simulink model "HLC_test_2018"  (R2020a)
settings: Solver=VariableStepAuto  StartTime=0.0  StopTime=10.0  RelTol=1e-3
values from neighbouring files (symbols this model uses):
  Ignition = timeseries    [TT1_in.m]
undefined symbols (not defined in the file or in its folder): Ambiant_Angle, DN, Light, Lock, Road_T, Speed_InKMPH, V_Detected, Weather
libraries: simulink x59
settings Model: Creator=VIJAY BANDEPPA MURGE  LastModifiedBy=VIJAY BANDEPPA MURGE
settings DebuggingCC: ArithmeticOperatorsInVariantConditions=warning
settings SFSimCC: CustomCodeUndefinedFunction=UseInterfaceOnly

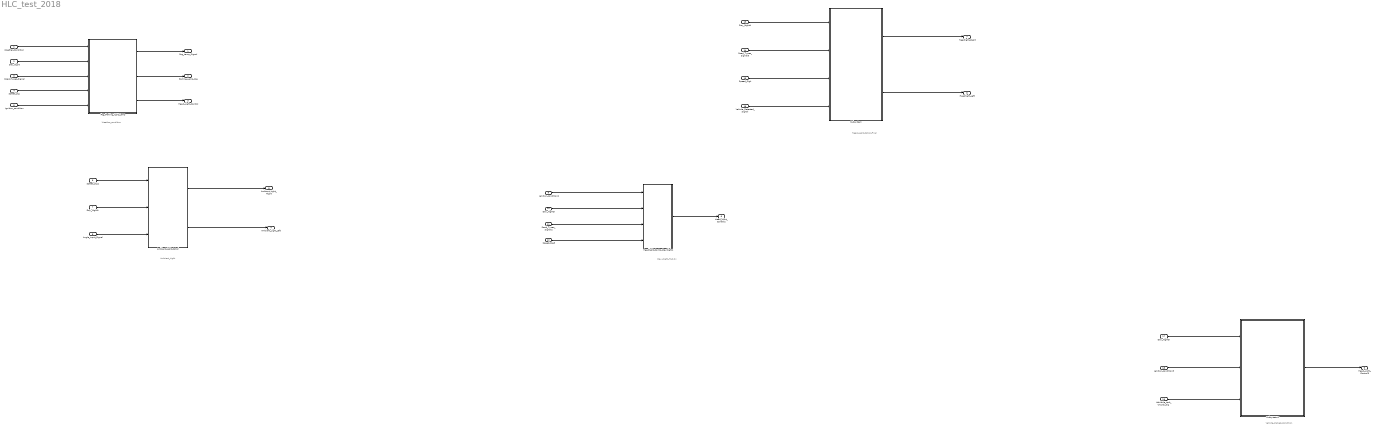
== system HLC_test_2018 ==
  note: Ambient_Light
  note: Day_Night_HLC.slx
  note: Head_Light_Cotrol_Final
  note: Vehicle_Parked_Condition
  note: Weather_condition
  Weather_Condition : Inport
  Day_Night : Inport  Port=2
  Road_Types_Signal : Inport  Port=3
  Speed_Sig : Inport  Port=4
  Ignition_condition : Inport  Port=5
  Speed_Sig1 : Inport  Port=6
  Day_Night1 : Inport  Port=7
  Angle_Input_Signal : Inport  Port=8
  Ignition_condition2 : Inport  Port=9
  Day_Night3 : Inport  Port=10
  Road_Types_Signal2 : Inport  Port=11
  Speed_Sig3 : Inport  Port=12
  Day_Night4 : Inport  Port=13
  Road_Types_Signal3 : Inport  Port=14
  Speed_Sig4 : Inport  Port=15
  Vehicle_Detected_Signal : Inport  Port=16
  Day_Night5 : Inport  Port=17
  Ignition_condition3 : Inport  Port=18
  Vehichle_Lock_UnLock_Sig : Inport  Port=19
  Ambient_Light_Cotrol : Subsystem  Description=This System is use for cotrol abbiant Light Of cars and other havey loded vehicles
  Fog_Parking_light_Lamp : Subsystem  Description=Cotrol of Fog lamp_Parking Light and hedlight in differant modes
  Headlight_Contro_DayNight1 : Subsystem  Description=testing_dayNight_Control of the cars
  Subsystem : Subsystem
  Subsystem2 : Subsystem
  Fog_Lamp_Signal : Outport
  Parking_Lamp_Sig : Outport  Port=2
  Head_Light_Control : Outport  Port=3
  Ambiant_Light_Left : Outport  Port=4
  Ambiant_Light_Right : Outport  Port=5
  Head_Light_Control2 : Outport  Port=6
  Headlight_Right : Outport  Port=7
  Headlight_Left : Outport  Port=8
  Head_Light_Control3 : Outport  Port=9
  wires:
  Fog_Parking_light_Lamp/3(Head_Light_Control) -> Head_Light_Control/1
  Ignition_condition/1 -> Fog_Parking_light_Lamp/5(Ignition_condition)  "Ignition_condition"
  Fog_Parking_light_Lamp/2(Parking_Lamp_Sig) -> Parking_Lamp_Sig/1
  Weather_Condition/1 -> Fog_Parking_light_Lamp/1(Weather_Condition)  "Weather_Condition"
  Fog_Parking_light_Lamp/1(Fog_Lamp_Signal) -> Fog_Lamp_Signal/1
  Speed_Sig/1 -> Fog_Parking_light_Lamp/4(Speed_Sig)  "Speed_Sig"
  Day_Night/1 -> Fog_Parking_light_Lamp/2(Day_Night)  "Day_Night"
  Road_Types_Signal/1 -> Fog_Parking_light_Lamp/3(Road_Types_Signal)  "Road_Types_Signal"
  Day_Night1/1 -> Ambient_Light_Cotrol/2(Day_Night)  "Day_Night"
  Ambient_Light_Cotrol/1(Ambiant_Light_Right) -> Ambiant_Light_Right/1
  Angle_Input_Signal/1 -> Ambient_Light_Cotrol/3(Angle_Input_Signal)  "Angle_Input_Signal"
  Speed_Sig1/1 -> Ambient_Light_Cotrol/1(Speed_Sig)  "Speed_Sig"
  Ambient_Light_Cotrol/2(Ambiant_Light_Left) -> Ambiant_Light_Left/1
  Ignition_condition2/1 -> Headlight_Contro_DayNight1/1(Ignition_condition)  "Ignition_condition"
  Day_Night3/1 -> Headlight_Contro_DayNight1/2(Day_Night)  "Day_Night"
  Speed_Sig3/1 -> Headlight_Contro_DayNight1/4(Speed_Sig)  "Speed_Sig"
  Headlight_Contro_DayNight1/1(Head_Light_Control) -> Head_Light_Control2/1
  Road_Types_Signal2/1 -> Headlight_Contro_DayNight1/3(Road_Types_Signal)  "Road_Types_Signal"
  Speed_Sig4/1 -> Subsystem/3(Speed_Sig)  "Speed_Sig"
  Road_Types_Signal3/1 -> Subsystem/2(Road_Types_Signal)  "Road_Types_Signal"
  Vehicle_Detected_Signal/1 -> Subsystem/4(Vehicle_Detected_Signal)  "Vehicle_Detected_Signal"
  Subsystem/1(Headlight_Right) -> Headlight_Right/1
  Subsystem/2(Headlight_Left) -> Headlight_Left/1
  Day_Night4/1 -> Subsystem/1(Day_Night)  "Day_Night"
  Subsystem2/1(Head_Light_Control) -> Head_Light_Control3/1
  Vehichle_Lock_UnLock_Sig/1 -> Subsystem2/3(Vehichle_Lock_UnLock_Sig)  "Vehichle_Lock_UnLock_Sig"
  Ignition_condition3/1 -> Subsystem2/2(Ignition_condition)  "Ignition_condition"
  Day_Night5/1 -> Subsystem2/1(Day_Night)  "Day_Night"

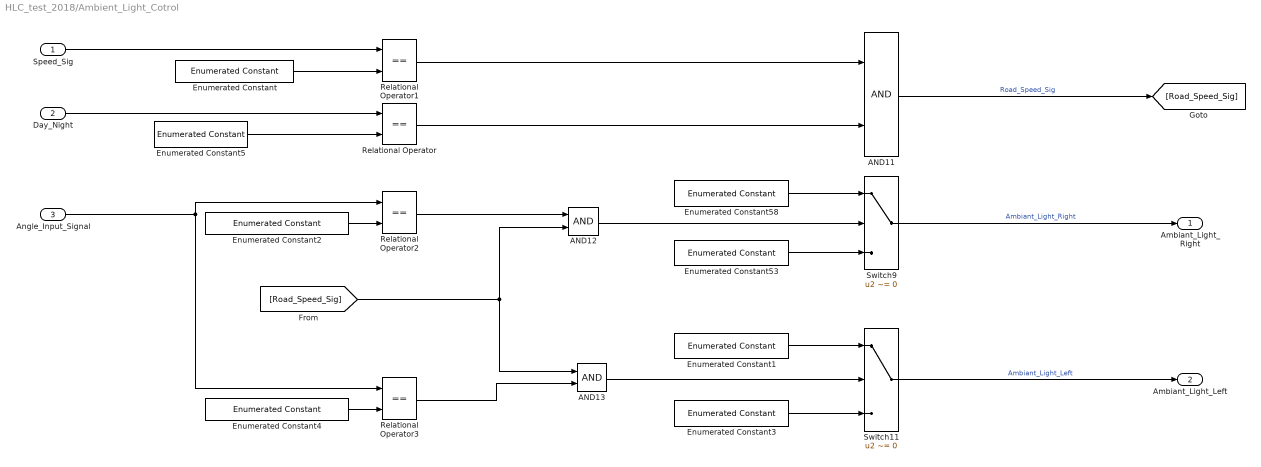
== system HLC_test_2018/Ambient_Light_Cotrol ==
  Speed_Sig : Inport
  Day_Night : Inport  Port=2
  Angle_Input_Signal : Inport  Port=3
  AND11 : Logic  AllPortsSameDT=off
  AND12 : Logic  AllPortsSameDT=off
  AND13 : Logic  AllPortsSameDT=off
  Enumerated Constant : simulink/Sources/Enumerated Constant  OutDataTypeStr=Enum: Speed_InKMPH  Value=Speed_InKMPH.Speed_Value  SampleTime=inf
  Enumerated Constant1 : simulink/Sources/Enumerated Constant  OutDataTypeStr=Enum: Light  Value=Light.L_Ambient_Light_On  SampleTime=inf
  Enumerated Constant2 : simulink/Sources/Enumerated Constant  OutDataTypeStr=Enum: Ambiant_Angle  Value=Ambiant_Angle.Ambiant_RHS_Angle  SampleTime=inf
  Enumerated Constant3 : simulink/Sources/Enumerated Constant  OutDataTypeStr=Enum: Light  Value=Light.L_Ambient_Light_off  SampleTime=inf
  Enumerated Constant4 : simulink/Sources/Enumerated Constant  OutDataTypeStr=Enum: Ambiant_Angle  Value=Ambiant_Angle.Ambiant_LHS_Angle  SampleTime=inf
  Enumerated Constant5 : simulink/Sources/Enumerated Constant  OutDataTypeStr=Enum: DN  Value=DN.Darkness  SampleTime=inf
  Enumerated Constant53 : simulink/Sources/Enumerated Constant  OutDataTypeStr=Enum: Light  Value=Light.R_Ambient_Light_off  SampleTime=inf
  Enumerated Constant58 : simulink/Sources/Enumerated Constant  OutDataTypeStr=Enum: Light  Value=Light.R_Ambient_Light_On  SampleTime=inf
  Relational Operator : RelationalOperator  Operator===  OutDataTypeStr=boolean  RndMeth=Simplest
  Relational Operator1 : RelationalOperator  Operator===  OutDataTypeStr=boolean  RndMeth=Simplest
  Relational Operator2 : RelationalOperator  Operator===  OutDataTypeStr=boolean  RndMeth=Simplest
  Relational Operator3 : RelationalOperator  Operator===  RndMeth=Simplest
  Switch11 : Switch  Criteria=u2 ~= 0  OutDataTypeStr=Inherit: Inherit via back propagation
  Switch9 : Switch  Criteria=u2 ~= 0  OutDataTypeStr=Inherit: Inherit via back propagation
  Ambiant_Light_Right : Outport
  Ambiant_Light_Left : Outport  Port=2
  wires:
  Enumerated Constant5/1 -> Relational Operator/2
  [Road_Speed_Sig] -> AND12/2, AND13/1
  Angle_Input_Signal/1 -> Relational Operator2/1, Relational Operator3/1
  Relational Operator3/1 -> AND13/2
  AND11/1 -> [Road_Speed_Sig]  "Road_Speed_Sig"
  AND12/1 -> Switch9/2
  Enumerated Constant1/1 -> Switch11/1
  AND13/1 -> Switch11/2
  Enumerated Constant58/1 -> Switch9/1
  Relational Operator2/1 -> AND12/1
  Relational Operator/1 -> AND11/2
  Enumerated Constant53/1 -> Switch9/3
  Enumerated Constant3/1 -> Switch11/3
  Day_Night/1 -> Relational Operator/1
  Switch9/1 -> Ambiant_Light_Right/1  "Ambiant_Light_Right"
  Switch11/1 -> Ambiant_Light_Left/1  "Ambiant_Light_Left"
  Speed_Sig/1 -> Relational Operator1/1
  Enumerated Constant/1 -> Relational Operator1/2
  Relational Operator1/1 -> AND11/1
  Enumerated Constant2/1 -> Relational Operator2/2
  Enumerated Constant4/1 -> Relational Operator3/2

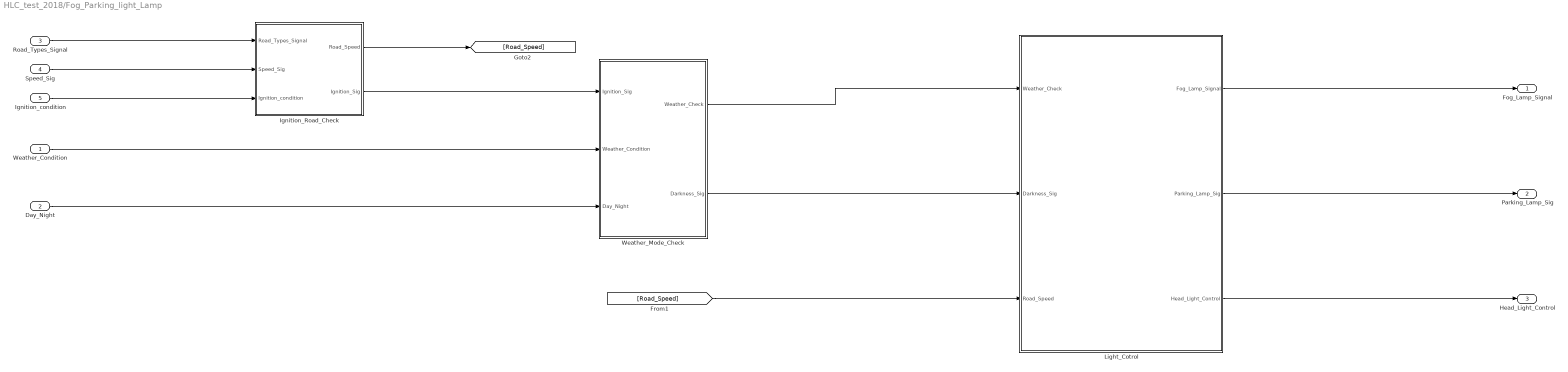
== system HLC_test_2018/Fog_Parking_light_Lamp ==
  Weather_Condition : Inport
  Day_Night : Inport  Port=2
  Road_Types_Signal : Inport  Port=3
  Speed_Sig : Inport  Port=4
  Ignition_condition : Inport  Port=5
  Ignition_Road_Check : Subsystem  Description=ignition and Road_Check
  Light_Cotrol : Subsystem  Description=it control the fog parking and head light
  Weather_Mode_Check : Subsystem  Description=it check weather and raod conditions
  Fog_Lamp_Signal : Outport
  Parking_Lamp_Sig : Outport  Port=2
  Head_Light_Control : Outport  Port=3
  wires:
  Weather_Condition/1 -> Weather_Mode_Check/2(Weather_Condition)
  Ignition_Road_Check/2(Ignition_Sig) -> Weather_Mode_Check/1(Ignition_Sig)
  Day_Night/1 -> Weather_Mode_Check/3(Day_Night)
  Road_Types_Signal/1 -> Ignition_Road_Check/1(Road_Types_Signal)
  Speed_Sig/1 -> Ignition_Road_Check/2(Speed_Sig)
  Ignition_condition/1 -> Ignition_Road_Check/3(Ignition_condition)
  Ignition_Road_Check/1(Road_Speed) -> [Road_Speed]
  Weather_Mode_Check/1(Weather_Check) -> Light_Cotrol/1(Weather_Check)
  Weather_Mode_Check/2(Darkness_Sig) -> Light_Cotrol/2(Darkness_Sig)
  Light_Cotrol/1(Fog_Lamp_Signal) -> Fog_Lamp_Signal/1
  Light_Cotrol/2(Parking_Lamp_Sig) -> Parking_Lamp_Sig/1
  Light_Cotrol/3(Head_Light_Control) -> Head_Light_Control/1
  [Road_Speed] -> Light_Cotrol/3(Road_Speed)

== system HLC_test_2018/Headlight_Contro_DayNight1 ==
  Ignition_condition : Inport
  Day_Night : Inport  Port=2
  Road_Types_Signal : Inport  Port=3
  Speed_Sig : Inport  Port=4
  Day_Ignition_Check : Subsystem  Description=check road and ignition condition
  Road_Syateam : Subsystem  Description=Road check condition
  Head_Light_Control : Outport
  wires:
  Road_Types_Signal/1 -> Road_Syateam/1(Road_Types_Signal)
  Speed_Sig/1 -> Road_Syateam/2(Speed_Sig)
  Ignition_condition/1 -> Day_Ignition_Check/1(Ignition_condition)
  Day_Night/1 -> Day_Ignition_Check/2(Day_Night)
  Day_Ignition_Check/1(Head_Light_Control) -> Head_Light_Control/1
  Road_Syateam/1(Road_Speed_Signal_Check) -> Day_Ignition_Check/3(Road_Speed_Signal_Check)

== system HLC_test_2018/Subsystem ==
  Day_Night : Inport
  Road_Types_Signal : Inport  Port=2
  Speed_Sig : Inport  Port=3
  Vehicle_Detected_Signal : Inport  Port=4
  Head_Light_Cotrol : Subsystem
  RHS_LHS_Vehicle_Detct : Subsystem
  Road_Vehicle_Dect : Subsystem
  Headlight_Right : Outport
  Headlight_Left : Outport  Port=2
  wires:
  Road_Types_Signal/1 -> Road_Vehicle_Dect/1(Road_Types_Signal)
  Speed_Sig/1 -> Road_Vehicle_Dect/2(Speed_Sig)
  Vehicle_Detected_Signal/1 -> RHS_LHS_Vehicle_Detct/1(Vehicle_Detected_Signal), Road_Vehicle_Dect/3(Vehicle_Detected_Signal)
  [Day_Night] -> RHS_LHS_Vehicle_Detct/2(Day_Night)
  Day_Night/1 -> [Day_Night], Head_Light_Cotrol/1(Day_Night)
  Road_Vehicle_Dect/1(Road_Vehical_Signal) -> Head_Light_Cotrol/2(Road_Vehical_Signal)
  RHS_LHS_Vehicle_Detct/1(Right_Vehicle_Detected) -> Head_Light_Cotrol/3(Right_Vehicle_Detected)
  RHS_LHS_Vehicle_Detct/2(Left_Vehicle_Detected) -> Head_Light_Cotrol/4(Left_Vehicle_Detected)
  Head_Light_Cotrol/1(Headlight_Right) -> Headlight_Right/1
  Head_Light_Cotrol/2(Headlight_Left) -> Headlight_Left/1

== system HLC_test_2018/Subsystem2 ==
  Day_Night : Inport
  Ignition_condition : Inport  Port=2
  Vehichle_Lock_UnLock_Sig : Inport  Port=3
  Subsystem : Subsystem
  Subsystem1 : Subsystem
  Head_Light_Control : Outport
  wires:
  Subsystem/5(Lock_Sig) -> Subsystem1/5(Lock_Sig)
  Subsystem/4(Ignition_sig) -> Subsystem1/4(Ignition_sig)
  Subsystem/1(Day_Night_Sig) -> Subsystem1/1(Day_Night_Sig)
  Subsystem/2(Day_Ign_Lock_Sig) -> Subsystem1/2(Day_Ign_Lock_Sig)
  Subsystem/3(Darkness_Sig) -> Subsystem1/3(Darkness_Sig)
  Day_Night/1 -> Subsystem/1(Day_Night)
  Subsystem1/1(Head_Light_Control) -> Head_Light_Control/1
  Ignition_condition/1 -> Subsystem/2(Ignition_condition)
  Vehichle_Lock_UnLock_Sig/1 -> Subsystem/3(Vehichle_Lock_UnLock_Sig)

== system HLC_test_2018/Fog_Parking_light_Lamp/Ignition_Road_Check ==
  Road_Types_Signal : Inport
  Speed_Sig : Inport  Port=2
  Ignition_condition : Inport  Port=3
  AND9 : Logic  Inputs=3  AllPortsSameDT=off  OutDataTypeStr=boolean
  Compare To Constant : simulink/Logic and Bit Operations/Compare To Constant  relop=<=  const=3.0  OutDataTypeStr=boolean
  Enumerated Constant54 : simulink/Sources/Enumerated Constant  OutDataTypeStr=Enum: Ignition  Value=Ignition.Ignition_On  SampleTime=inf
  Enumerated Constant6 : simulink/Sources/Enumerated Constant  OutDataTypeStr=Enum: Road_T  Value=Road_T.Inside_City_Road  SampleTime=inf
  Relational Operator1 : RelationalOperator  Operator=~=  OutDataTypeStr=boolean  RndMeth=Simplest
  Relational Operator18 : RelationalOperator  Operator===  OutDataTypeStr=boolean  RndMeth=Simplest
  Road_Speed : Outport
  Ignition_Sig : Outport  Port=2
  wires:
  Enumerated Constant6/1 -> Relational Operator1/2
  Relational Operator18/1 -> Ignition_Sig/1, AND9/3  "Ignition_Sig"
  Relational Operator1/1 -> AND9/1
  Enumerated Constant54/1 -> Relational Operator18/2
  Compare To Constant/1 -> AND9/2
  AND9/1 -> Road_Speed/1  "Road_Speed"
  Speed_Sig/1 -> Compare To Constant/1
  Road_Types_Signal/1 -> Relational Operator1/1
  Ignition_condition/1 -> Relational Operator18/1

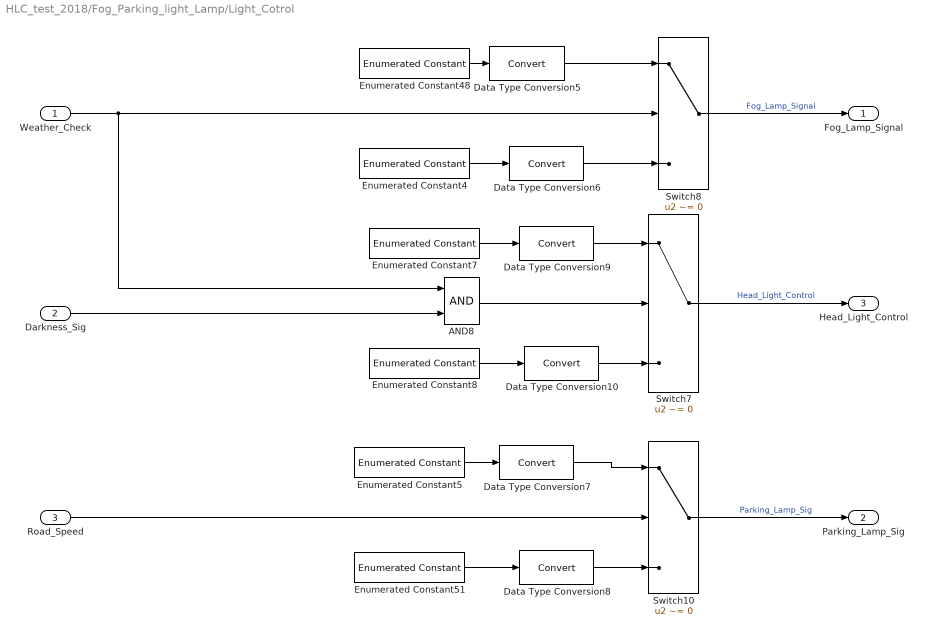
== system HLC_test_2018/Fog_Parking_light_Lamp/Light_Cotrol ==
  Weather_Check : Inport
  Darkness_Sig : Inport  Port=2
  Road_Speed : Inport  Port=3
  AND8 : Logic  AllPortsSameDT=off  OutDataTypeStr=boolean
  Data Type Conversion{5..10} (6 alike) : DataTypeConversion
  Enumerated Constant4 : simulink/Sources/Enumerated Constant  OutDataTypeStr=Enum: Light  Value=Light.Fog_Lamp_off  SampleTime=inf
  Enumerated Constant48 : simulink/Sources/Enumerated Constant  OutDataTypeStr=Enum: Light  Value=Light.Fog_Lamp_ON  SampleTime=inf
  Enumerated Constant5 : simulink/Sources/Enumerated Constant  OutDataTypeStr=Enum: Light  Value=Light.Parking_Light_On  SampleTime=inf
  Enumerated Constant51 : simulink/Sources/Enumerated Constant  OutDataTypeStr=Enum: Light  Value=Light.Parking_Light_Off  SampleTime=inf
  Enumerated Constant7 : simulink/Sources/Enumerated Constant  OutDataTypeStr=Enum: Light  Value=Light.Low_Beam  SampleTime=inf
  Enumerated Constant8 : simulink/Sources/Enumerated Constant  OutDataTypeStr=Enum: Light  Value=Light.Headlight_Off  SampleTime=inf
  Switch10 : Switch  Criteria=u2 ~= 0  OutDataTypeStr=Inherit: Inherit via back propagation
  Switch7 : Switch  Criteria=u2 ~= 0  OutDataTypeStr=Inherit: Inherit via back propagation
  Switch8 : Switch  Criteria=u2 ~= 0  OutDataTypeStr=Inherit: Inherit via back propagation
  Fog_Lamp_Signal : Outport
  Parking_Lamp_Sig : Outport  Port=2
  Head_Light_Control : Outport  Port=3
  wires:
  Enumerated Constant48/1 -> Data Type Conversion5/1
  Enumerated Constant51/1 -> Data Type Conversion8/1
  Data Type Conversion10/1 -> Switch7/3
  Data Type Conversion7/1 -> Switch10/1
  AND8/1 -> Switch7/2
  Data Type Conversion9/1 -> Switch7/1
  Enumerated Constant4/1 -> Data Type Conversion6/1
  Data Type Conversion5/1 -> Switch8/1
  Enumerated Constant8/1 -> Data Type Conversion10/1
  Enumerated Constant7/1 -> Data Type Conversion9/1
  Data Type Conversion8/1 -> Switch10/3
  Enumerated Constant5/1 -> Data Type Conversion7/1
  Data Type Conversion6/1 -> Switch8/3
  Weather_Check/1 -> AND8/1, Switch8/2
  Road_Speed/1 -> Switch10/2
  Switch10/1 -> Parking_Lamp_Sig/1  "Parking_Lamp_Sig"
  Switch8/1 -> Fog_Lamp_Signal/1  "Fog_Lamp_Signal"
  Darkness_Sig/1 -> AND8/2
  Switch7/1 -> Head_Light_Control/1  "Head_Light_Control"

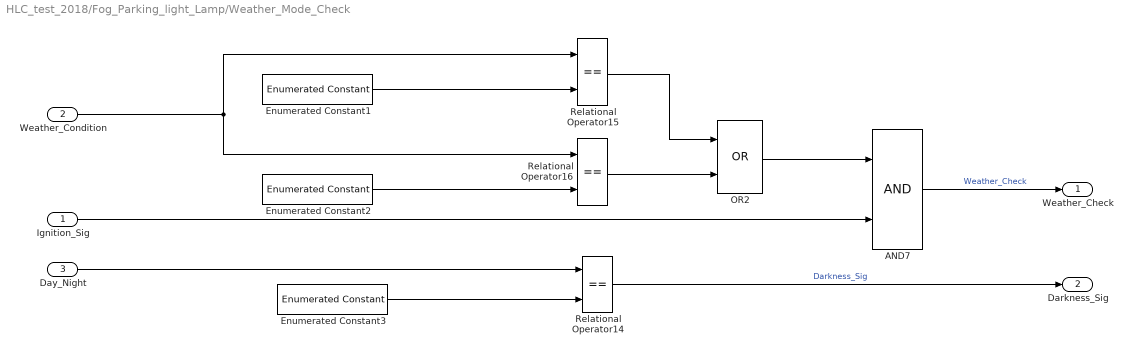
== system HLC_test_2018/Fog_Parking_light_Lamp/Weather_Mode_Check ==
  Ignition_Sig : Inport
  Weather_Condition : Inport  Port=2
  Day_Night : Inport  Port=3
  AND7 : Logic  AllPortsSameDT=off  OutDataTypeStr=boolean
  Enumerated Constant1 : simulink/Sources/Enumerated Constant  OutDataTypeStr=Enum: Weather  Value=Weather.Fog_Detected  SampleTime=inf
  Enumerated Constant2 : simulink/Sources/Enumerated Constant  OutDataTypeStr=Enum: Weather  Value=Weather.Rain_Detected  SampleTime=inf
  Enumerated Constant3 : simulink/Sources/Enumerated Constant  OutDataTypeStr=Enum: DN  Value=DN.Darkness  SampleTime=inf
  OR2 : Logic  Operator=OR  AllPortsSameDT=off  OutDataTypeStr=boolean
  Relational Operator14 : RelationalOperator  Operator===  OutDataTypeStr=boolean  RndMeth=Simplest
  Relational Operator15 : RelationalOperator  Operator===  OutDataTypeStr=boolean  RndMeth=Simplest
  Relational Operator16 : RelationalOperator  Operator===  OutDataTypeStr=boolean  RndMeth=Simplest
  Weather_Check : Outport
  Darkness_Sig : Outport  Port=2
  wires:
  Ignition_Sig/1 -> AND7/2
  Enumerated Constant2/1 -> Relational Operator16/2
  Weather_Condition/1 -> Relational Operator15/1, Relational Operator16/1
  Enumerated Constant3/1 -> Relational Operator14/2
  Enumerated Constant1/1 -> Relational Operator15/2
  Relational Operator15/1 -> OR2/1
  OR2/1 -> AND7/1
  Relational Operator16/1 -> OR2/2
  AND7/1 -> Weather_Check/1  "Weather_Check"
  Day_Night/1 -> Relational Operator14/1
  Relational Operator14/1 -> Darkness_Sig/1  "Darkness_Sig"

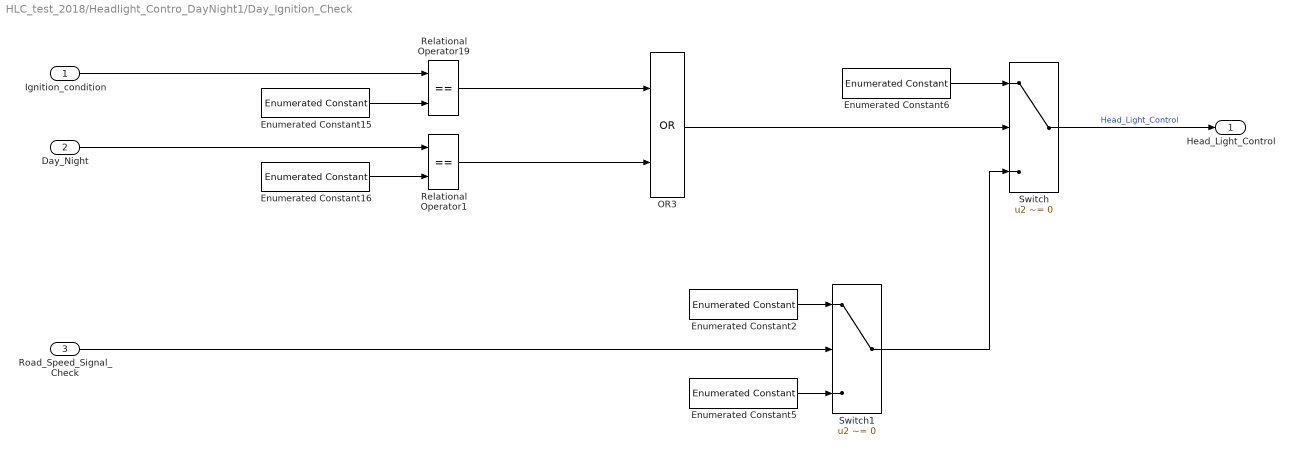
== system HLC_test_2018/Headlight_Contro_DayNight1/Day_Ignition_Check ==
  Ignition_condition : Inport
  Day_Night : Inport  Port=2
  Road_Speed_Signal_Check : Inport  Port=3
  Enumerated Constant15 : simulink/Sources/Enumerated Constant  OutDataTypeStr=Enum: Ignition  Value=Ignition.Ignition_Off  SampleTime=inf
  Enumerated Constant16 : simulink/Sources/Enumerated Constant  OutDataTypeStr=Enum: DN  Value=DN.Day_Time  SampleTime=inf
  Enumerated Constant2 : simulink/Sources/Enumerated Constant  OutDataTypeStr=Enum: Light  Value=Light.High_beam  SampleTime=inf
  Enumerated Constant5 : simulink/Sources/Enumerated Constant  OutDataTypeStr=Enum: Light  Value=Light.Low_Beam  SampleTime=inf
  Enumerated Constant6 : simulink/Sources/Enumerated Constant  OutDataTypeStr=Enum: Light  Value=Light.Headlight_Off  SampleTime=inf
  OR3 : Logic  Operator=OR  AllPortsSameDT=off  OutDataTypeStr=boolean
  Relational Operator1 : RelationalOperator  Operator===  OutDataTypeStr=boolean  RndMeth=Simplest
  Relational Operator19 : RelationalOperator  Operator===  OutDataTypeStr=boolean  RndMeth=Simplest
  Switch : Switch  Criteria=u2 ~= 0  OutDataTypeStr=Inherit: Inherit via back propagation
  Switch1 : Switch  Criteria=u2 ~= 0
  Head_Light_Control : Outport
  wires:
  Enumerated Constant6/1 -> Switch/1
  OR3/1 -> Switch/2
  Switch1/1 -> Switch/3
  Relational Operator19/1 -> OR3/1
  Enumerated Constant16/1 -> Relational Operator1/2
  Relational Operator1/1 -> OR3/2
  Enumerated Constant2/1 -> Switch1/1
  Enumerated Constant5/1 -> Switch1/3
  Enumerated Constant15/1 -> Relational Operator19/2
  Road_Speed_Signal_Check/1 -> Switch1/2
  Switch/1 -> Head_Light_Control/1  "Head_Light_Control"
  Ignition_condition/1 -> Relational Operator19/1
  Day_Night/1 -> Relational Operator1/1

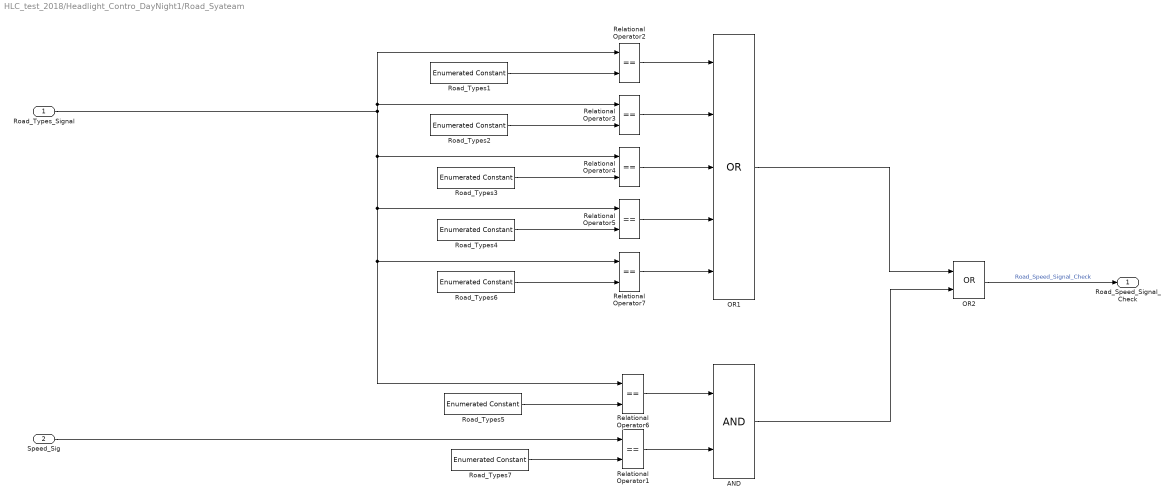
== system HLC_test_2018/Headlight_Contro_DayNight1/Road_Syateam ==
  Road_Types_Signal : Inport
  Speed_Sig : Inport  Port=2
  AND : Logic  AllPortsSameDT=off  OutDataTypeStr=boolean
  OR1 : Logic  Operator=OR  Inputs=5  AllPortsSameDT=off  OutDataTypeStr=boolean
  OR2 : Logic  Operator=OR  AllPortsSameDT=off  OutDataTypeStr=boolean
  Relational Operator{1..7} (7 alike) : RelationalOperator  Operator===  OutDataTypeStr=boolean  RndMeth=Simplest
  Road_Types1 : simulink/Sources/Enumerated Constant  OutDataTypeStr=Enum: Road_T  Value=Road_T.Express_Way  SampleTime=inf
  Road_Types2 : simulink/Sources/Enumerated Constant  OutDataTypeStr=Enum: Road_T  Value=Road_T.High_Way  SampleTime=inf
  Road_Types3 : simulink/Sources/Enumerated Constant  OutDataTypeStr=Enum: Road_T  Value=Road_T.Rural_Road  SampleTime=inf
  Road_Types4 : simulink/Sources/Enumerated Constant  OutDataTypeStr=Enum: Road_T  Value=Road_T.Outside_City_Road  SampleTime=inf
  Road_Types5 : simulink/Sources/Enumerated Constant  OutDataTypeStr=Enum: Road_T  Value=Road_T.Inside_City_Road  SampleTime=inf
  Road_Types6 : simulink/Sources/Enumerated Constant  OutDataTypeStr=Enum: Road_T  Value=Road_T.Tunnel_Road  SampleTime=inf
  Road_Types7 : simulink/Sources/Enumerated Constant  OutDataTypeStr=Enum: Speed_InKMPH  Value=Speed_InKMPH.Speed_Value  SampleTime=inf
  Road_Speed_Signal_Check : Outport
  wires:
  Relational Operator4/1 -> OR1/3
  OR1/1 -> OR2/1
  Speed_Sig/1 -> Relational Operator1/1
  Relational Operator7/1 -> OR1/5
  Road_Types3/1 -> Relational Operator4/2
  Relational Operator3/1 -> OR1/2
  Road_Types_Signal/1 -> Relational Operator6/1, Relational Operator7/1, Relational Operator5/1, Relational Operator4/1, Relational Operator3/1, Relational Operator2/1
  Relational Operator6/1 -> AND/1
  AND/1 -> OR2/2
  Relational Operator2/1 -> OR1/1
  Road_Types5/1 -> Relational Operator6/2
  Road_Types2/1 -> Relational Operator3/2
  Road_Types4/1 -> Relational Operator5/2
  Road_Types6/1 -> Relational Operator7/2
  Road_Types1/1 -> Relational Operator2/2
  Relational Operator1/1 -> AND/2
  Relational Operator5/1 -> OR1/4
  OR2/1 -> Road_Speed_Signal_Check/1  "Road_Speed_Signal_Check"
  Road_Types7/1 -> Relational Operator1/2

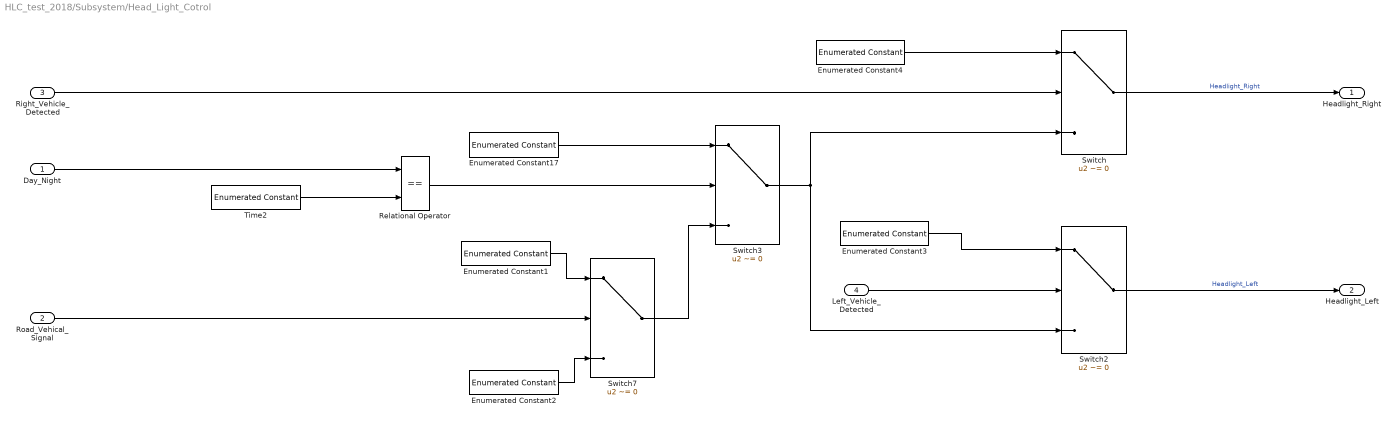
== system HLC_test_2018/Subsystem/Head_Light_Cotrol ==
  Day_Night : Inport
  Road_Vehical_Signal : Inport  Port=2
  Right_Vehicle_Detected : Inport  Port=3
  Left_Vehicle_Detected : Inport  Port=4
  Enumerated Constant1 : simulink/Sources/Enumerated Constant  OutDataTypeStr=Enum: Light  Value=Light.High_beam  SampleTime=inf
  Enumerated Constant17 : simulink/Sources/Enumerated Constant  OutDataTypeStr=Enum: Light  Value=Light.Headlight_Off  SampleTime=inf
  Enumerated Constant2 : simulink/Sources/Enumerated Constant  OutDataTypeStr=Enum: Light  Value=Light.Low_Beam  SampleTime=inf
  Enumerated Constant3 : simulink/Sources/Enumerated Constant  OutDataTypeStr=Enum: Light  Value=Light.Low_Beam  SampleTime=inf
  Enumerated Constant4 : simulink/Sources/Enumerated Constant  OutDataTypeStr=Enum: Light  Value=Light.Low_Beam  SampleTime=inf
  Relational Operator : RelationalOperator  Operator===  OutDataTypeStr=boolean  RndMeth=Simplest
  Switch : Switch  Criteria=u2 ~= 0  OutDataTypeStr=Inherit: Inherit via back propagation
  Switch2 : Switch  Criteria=u2 ~= 0  OutDataTypeStr=Inherit: Inherit via back propagation
  Switch3 : Switch  Criteria=u2 ~= 0
  Switch7 : Switch  Criteria=u2 ~= 0
  Time2 : simulink/Sources/Enumerated Constant  OutDataTypeStr=Enum: DN  Value=DN.Day_Time  SampleTime=inf
  Headlight_Right : Outport
  Headlight_Left : Outport  Port=2
  wires:
  Enumerated Constant2/1 -> Switch7/3
  Switch7/1 -> Switch3/3
  Left_Vehicle_Detected/1 -> Switch2/2
  Switch3/1 -> Switch/3, Switch2/3
  Switch2/1 -> Headlight_Left/1  "Headlight_Left"
  Enumerated Constant3/1 -> Switch2/1
  Enumerated Constant17/1 -> Switch3/1
  Enumerated Constant4/1 -> Switch/1
  Enumerated Constant1/1 -> Switch7/1
  Relational Operator/1 -> Switch3/2
  Time2/1 -> Relational Operator/2
  Road_Vehical_Signal/1 -> Switch7/2
  Switch/1 -> Headlight_Right/1  "Headlight_Right"
  Right_Vehicle_Detected/1 -> Switch/2
  Day_Night/1 -> Relational Operator/1

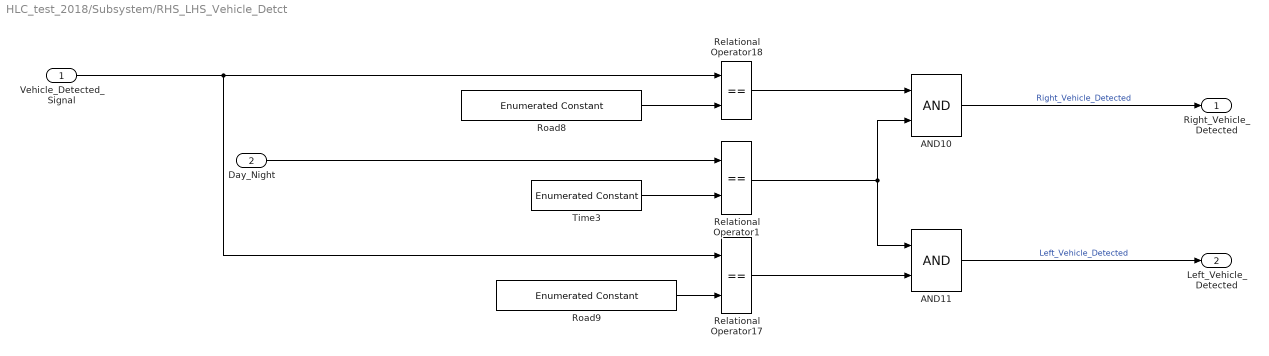
== system HLC_test_2018/Subsystem/RHS_LHS_Vehicle_Detct ==
  Vehicle_Detected_Signal : Inport
  Day_Night : Inport  Port=2
  AND10 : Logic  AllPortsSameDT=off  OutDataTypeStr=boolean
  AND11 : Logic  AllPortsSameDT=off  OutDataTypeStr=boolean
  Relational Operator1 : RelationalOperator  Operator===  OutDataTypeStr=boolean  RndMeth=Simplest
  Relational Operator17 : RelationalOperator  Operator===  OutDataTypeStr=boolean  RndMeth=Simplest
  Relational Operator18 : RelationalOperator  Operator===  OutDataTypeStr=boolean  RndMeth=Simplest
  Road8 : simulink/Sources/Enumerated Constant  OutDataTypeStr=Enum: V_Detected  Value=V_Detected.Vehicle_Detected_Right  SampleTime=inf
  Road9 : simulink/Sources/Enumerated Constant  OutDataTypeStr=Enum: V_Detected  Value=V_Detected.Vehicle_Detected_Left  SampleTime=inf
  Time3 : simulink/Sources/Enumerated Constant  OutDataTypeStr=Enum: DN  Value=DN.Darkness  SampleTime=inf
  Right_Vehicle_Detected : Outport
  Left_Vehicle_Detected : Outport  Port=2
  wires:
  AND11/1 -> Left_Vehicle_Detected/1  "Left_Vehicle_Detected"
  Relational Operator1/1 -> AND10/2, AND11/1
  Relational Operator18/1 -> AND10/1
  Road8/1 -> Relational Operator18/2
  Time3/1 -> Relational Operator1/2
  Road9/1 -> Relational Operator17/2
  Relational Operator17/1 -> AND11/2
  Vehicle_Detected_Signal/1 -> Relational Operator17/1, Relational Operator18/1
  AND10/1 -> Right_Vehicle_Detected/1  "Right_Vehicle_Detected"
  Day_Night/1 -> Relational Operator1/1

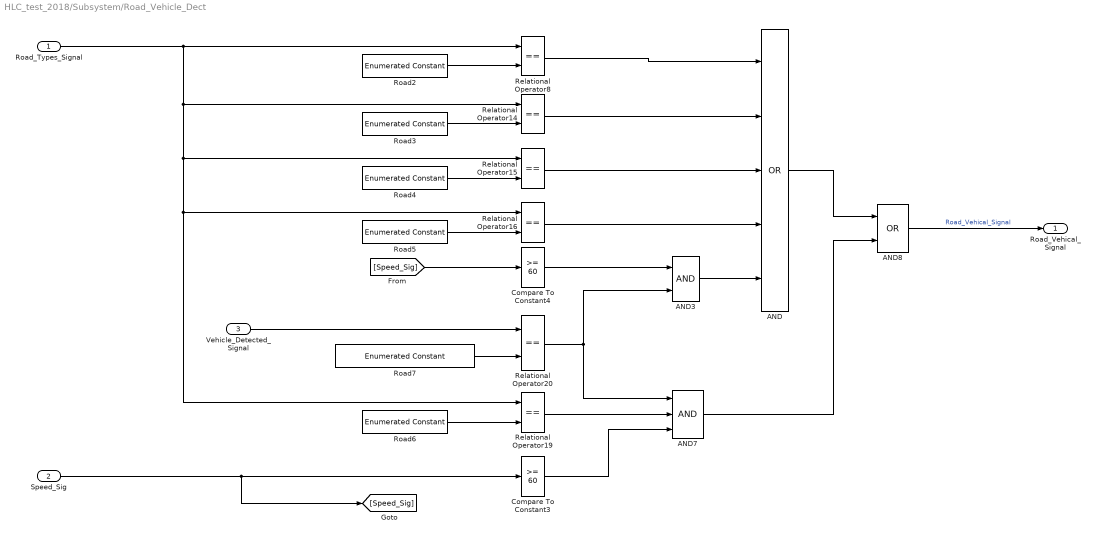
== system HLC_test_2018/Subsystem/Road_Vehicle_Dect ==
  Road_Types_Signal : Inport
  Speed_Sig : Inport  Port=2
  Vehicle_Detected_Signal : Inport  Port=3
  AND : Logic  Operator=OR  Inputs=5  AllPortsSameDT=off  OutDataTypeStr=boolean
  AND3 : Logic  AllPortsSameDT=off  OutDataTypeStr=boolean
  AND7 : Logic  Inputs=3  AllPortsSameDT=off  OutDataTypeStr=boolean
  AND8 : Logic  Operator=OR  AllPortsSameDT=off  OutDataTypeStr=boolean
  Compare To Constant3 : simulink/Logic and Bit Operations/Compare To Constant  relop=>=  const=60  OutDataTypeStr=boolean
  Compare To Constant4 : simulink/Logic and Bit Operations/Compare To Constant  relop=>=  const=60  OutDataTypeStr=boolean
  Relational Operator{8,14..16,19..20} (6 alike) : RelationalOperator  Operator===  OutDataTypeStr=boolean  RndMeth=Simplest
  Road2 : simulink/Sources/Enumerated Constant  OutDataTypeStr=Enum: Road_T  Value=Road_T.Express_Way  SampleTime=inf
  Road3 : simulink/Sources/Enumerated Constant  OutDataTypeStr=Enum: Road_T  Value=Road_T.High_Way  SampleTime=inf
  Road4 : simulink/Sources/Enumerated Constant  OutDataTypeStr=Enum: Road_T  Value=Road_T.Rural_Road  SampleTime=inf
  Road5 : simulink/Sources/Enumerated Constant  OutDataTypeStr=Enum: Road_T  Value=Road_T.Outside_City_Road  SampleTime=inf
  Road6 : simulink/Sources/Enumerated Constant  OutDataTypeStr=Enum: Road_T  Value=Road_T.Inside_City_Road  SampleTime=inf
  Road7 : simulink/Sources/Enumerated Constant  OutDataTypeStr=Enum: V_Detected  Value=V_Detected.No_Vehical_Detected  SampleTime=inf
  Road_Vehical_Signal : Outport
  wires:
  Road7/1 -> Relational Operator20/2
  Relational Operator20/1 -> AND7/1, AND3/2
  Road_Types_Signal/1 -> Relational Operator8/1, Relational Operator14/1, Relational Operator15/1, Relational Operator16/1, Relational Operator19/1
  Vehicle_Detected_Signal/1 -> Relational Operator20/1
  Speed_Sig/1 -> [Speed_Sig], Compare To Constant3/1
  Relational Operator15/1 -> AND/3
  Road2/1 -> Relational Operator8/2
  Road6/1 -> Relational Operator19/2
  Compare To Constant3/1 -> AND7/3
  Road5/1 -> Relational Operator16/2
  Road4/1 -> Relational Operator15/2
  Relational Operator16/1 -> AND/4
  Road3/1 -> Relational Operator14/2
  Relational Operator8/1 -> AND/1
  AND7/1 -> AND8/2
  Compare To Constant4/1 -> AND3/1
  Relational Operator14/1 -> AND/2
  Relational Operator19/1 -> AND7/2
  AND8/1 -> Road_Vehical_Signal/1  "Road_Vehical_Signal"
  AND/1 -> AND8/1
  AND3/1 -> AND/5
  [Speed_Sig] -> Compare To Constant4/1

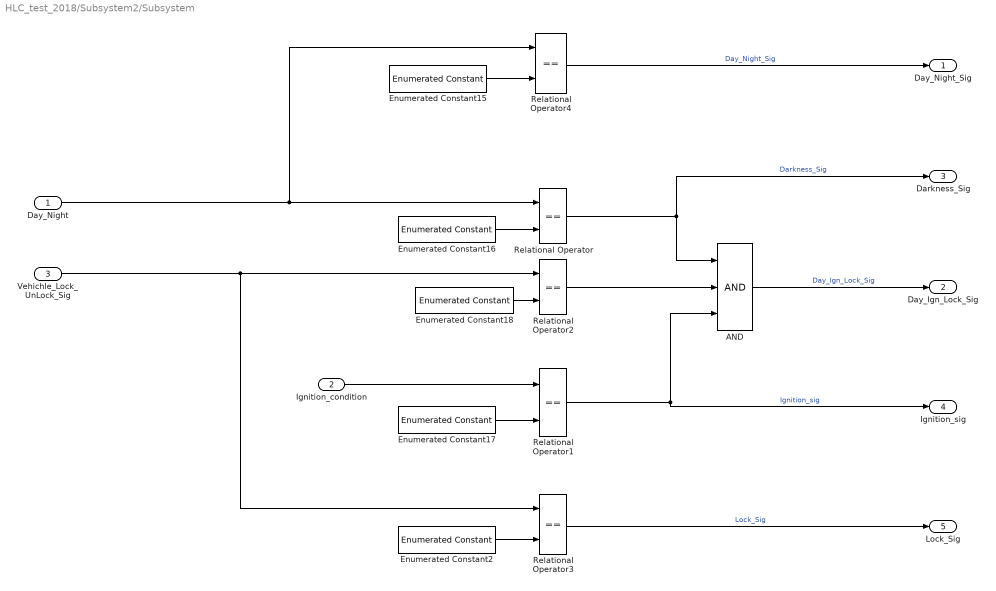
== system HLC_test_2018/Subsystem2/Subsystem ==
  Day_Night : Inport
  Ignition_condition : Inport  Port=2
  Vehichle_Lock_UnLock_Sig : Inport  Port=3
  AND : Logic  Inputs=3  AllPortsSameDT=off  OutDataTypeStr=boolean
  Enumerated Constant15 : simulink/Sources/Enumerated Constant  OutDataTypeStr=Enum: DN  Value=DN.Day_Time  SampleTime=inf
  Enumerated Constant16 : simulink/Sources/Enumerated Constant  OutDataTypeStr=Enum: DN  Value=DN.Darkness  SampleTime=inf
  Enumerated Constant17 : simulink/Sources/Enumerated Constant  OutDataTypeStr=Enum: Ignition  Value=Ignition.Ignition_Off  SampleTime=inf
  Enumerated Constant18 : simulink/Sources/Enumerated Constant  OutDataTypeStr=Enum: Lock  Value=Lock.Vehicle_locked  SampleTime=inf
  Enumerated Constant2 : simulink/Sources/Enumerated Constant  OutDataTypeStr=Enum: Lock  Value=Lock.Vehicle_locked  SampleTime=inf
  Relational Operator{,1..4} (5 alike) : RelationalOperator  Operator===  OutDataTypeStr=boolean  RndMeth=Simplest
  Day_Night_Sig : Outport
  Day_Ign_Lock_Sig : Outport  Port=2
  Darkness_Sig : Outport  Port=3
  Ignition_sig : Outport  Port=4
  Lock_Sig : Outport  Port=5
  wires:
  Enumerated Constant18/1 -> Relational Operator2/2
  Enumerated Constant16/1 -> Relational Operator/2
  Enumerated Constant2/1 -> Relational Operator3/2
  Enumerated Constant15/1 -> Relational Operator4/2
  Relational Operator1/1 -> AND/3, Ignition_sig/1  "Ignition_sig"
  Relational Operator/1 -> AND/1, Darkness_Sig/1  "Darkness_Sig"
  Vehichle_Lock_UnLock_Sig/1 -> Relational Operator2/1, Relational Operator3/1
  Day_Night/1 -> Relational Operator/1, Relational Operator4/1
  Enumerated Constant17/1 -> Relational Operator1/2
  AND/1 -> Day_Ign_Lock_Sig/1  "Day_Ign_Lock_Sig"
  Ignition_condition/1 -> Relational Operator1/1
  Relational Operator3/1 -> Lock_Sig/1  "Lock_Sig"
  Relational Operator4/1 -> Day_Night_Sig/1  "Day_Night_Sig"
  Relational Operator2/1 -> AND/2

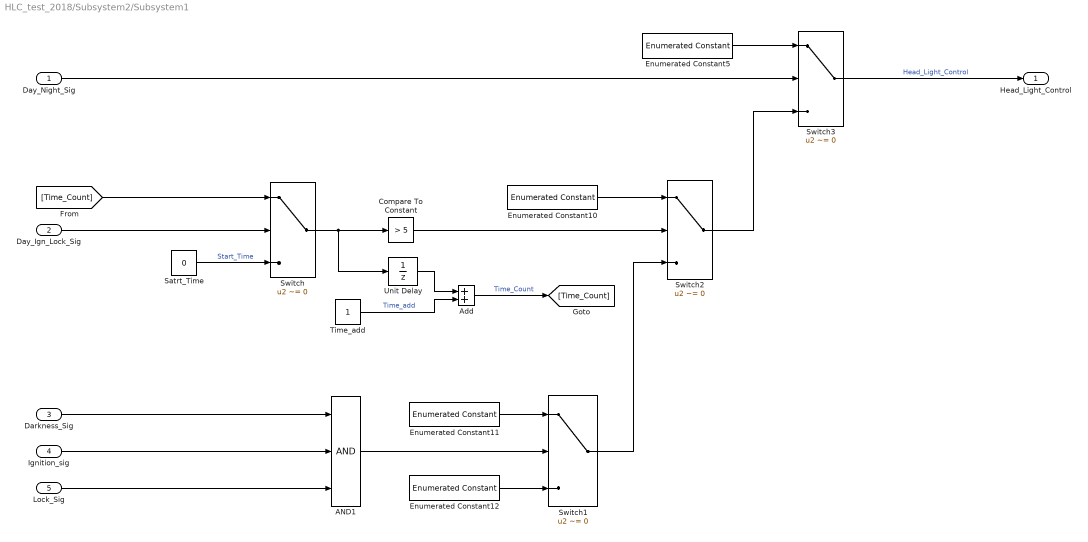
== system HLC_test_2018/Subsystem2/Subsystem1 ==
  Day_Night_Sig : Inport
  Day_Ign_Lock_Sig : Inport  Port=2
  Darkness_Sig : Inport  Port=3
  Ignition_sig : Inport  Port=4
  Lock_Sig : Inport  Port=5
  AND1 : Logic  Inputs=3  AllPortsSameDT=off  OutDataTypeStr=boolean
  Add : Sum
  Compare To Constant : simulink/Logic and Bit Operations/Compare To Constant  relop=>  const=5  OutDataTypeStr=boolean
  Enumerated Constant10 : simulink/Sources/Enumerated Constant  OutDataTypeStr=Enum: Light  Value=Light.Headlight_Off  SampleTime=inf
  Enumerated Constant11 : simulink/Sources/Enumerated Constant  OutDataTypeStr=Enum: Light  Value=Light.Low_Beam  SampleTime=inf
  Enumerated Constant12 : simulink/Sources/Enumerated Constant  OutDataTypeStr=Enum: Light  Value=Light.Low_Beam  SampleTime=inf
  Enumerated Constant5 : simulink/Sources/Enumerated Constant  OutDataTypeStr=Enum: Light  Value=Light.Headlight_Off  SampleTime=inf
  Satrt_Time : Constant  Value=0
  Switch : Switch  Criteria=u2 ~= 0
  Switch1 : Switch  Criteria=u2 ~= 0
  Switch2 : Switch  Criteria=u2 ~= 0
  Switch3 : Switch  Criteria=u2 ~= 0  OutDataTypeStr=Inherit: Inherit via back propagation
  Time_add : Constant
  Unit Delay : UnitDelay  SampleTime=-1  HasFrameUpgradeWarning=on
  Head_Light_Control : Outport
  wires:
  Enumerated Constant11/1 -> Switch1/1
  Day_Ign_Lock_Sig/1 -> Switch/2
  Day_Night_Sig/1 -> Switch3/2
  Switch1/1 -> Switch2/3
  Satrt_Time/1 -> Switch/3  "Start_Time"
  Darkness_Sig/1 -> AND1/1
  Switch2/1 -> Switch3/3
  Enumerated Constant12/1 -> Switch1/3
  Unit Delay/1 -> Add/1
  Enumerated Constant10/1 -> Switch2/1
  Enumerated Constant5/1 -> Switch3/1
  Time_add/1 -> Add/2  "Time_add"
  Lock_Sig/1 -> AND1/3
  Switch/1 -> Compare To Constant/1, Unit Delay/1
  AND1/1 -> Switch1/2
  Compare To Constant/1 -> Switch2/2
  Switch3/1 -> Head_Light_Control/1  "Head_Light_Control"
  Ignition_sig/1 -> AND1/2
  Add/1 -> [Time_Count]  "Time_Count"
  [Time_Count] -> Switch/1
